simulink model "motor_rotation"  (R2022a)
settings: Solver=VariableStepAuto  StartTime=0.0  StopTime=10.0  RelTol=1e-3  AbsTol=1e-3
libraries: fl_lib x26, nesl_utility x11, ee_lib x4, slpidlib x2
settings Model: Creator=venka  LastModifiedBy=venka
settings SolverCC: AutoScaleAbsTol=off  AlgebraicLoopSolver=TrustRegion
settings DebuggingCC: UnconnectedInputMsg=warning  UnconnectedOutputMsg=warning  UnconnectedLineMsg=warning  SymbolicDimsDataTypeCodeGenerationDiagnostic=none  SFMachineParentedDataDiag=warning
settings SFSimCC: CustomCodeUndefinedFunction=UseInterfaceOnly
settings RTWCC: DLArmComputeVersion=19.05
settings SimscapeCC: SimscapeLogType=all  SimscapeLogSimulationStatistics=on  SimscapeLogDataHistory=10000

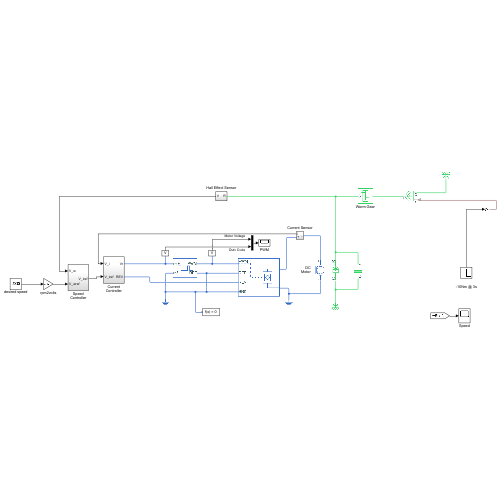
[thumbnail: Simulink's stored preview of the top-level diagram]
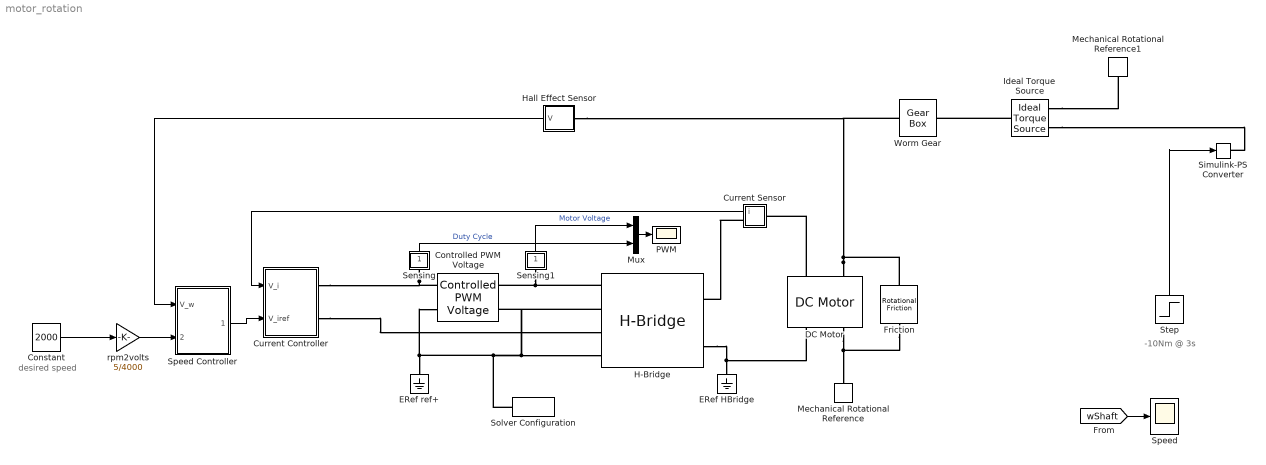
== system motor_rotation ==
  note: -10Nm @ 3s
  note: desired speed
  Constant : Constant  Value=2000
  Controlled PWM Voltage : ee_lib/Integrated Circuits/Controlled PWM Voltage  F=10000 Hz  TD=0 s  pulse_width_offset=0 s  pulse_min=0 s  pwm_or_av=2  event_type=1  sample_time=1e-6 s  Vmin=0 V  Vmax=5 V  Vm=5 V  u_min=0  u_max=1
  Current Controller : Subsystem
  Current Sensor : Subsystem
  DC Motor : ee_lib/Electromechanical/Brushed Motors/DC Motor  field_option=ee.enum.field_option.pm  Rf=100 Ohm  Lf=1 H  Laf=0.15 H  If0=0 A  parameterization=1  Ra=4.8 Ohm  La=1600e-6 H  emf_or_torque=2  Kv=0.0637 V/rpm  Ki=0.0637 N*m/A  T_stall=2.4e-4 N*m  w_max=1.91e+4 rpm  w_rated=1.5e+4 rpm  P_rated=0.08 W  V_rated=1.5 V  lam_param=1  i_noload=0 A  V_i_noload=1.5 V  J=2.5e-5 kg*m^2  lam=1e-08 N*m/(rad/s)  speed0=0 rpm  enable_fault_armature=simscape.enum.onoff.off  rev_faulted=1 / 3  G_faulted_armature=1e-5 S  fault_trigger_armature=ee.enum.faults.faultTrigger.temporal  t_fault_armature=1 s  max_permissible_current_armature=inf A  t_fail_on_current_armature=1 s  enable_fault_field=simscape.enum.onoff.off  G_faulted_field=1e-5 S  fault_trigger_field=ee.enum.faults.faultTrigger.temporal  t_fault_field=1 s  max_permissible_current_field=inf A  t_fail_on_current_field=1 s  fault_action=simscape.enum.assert.action.none  alpha=3.93e-3 1/K  Tmeas=25 degC  thermal_mass=100 J/K  initial_temperature=25 degC
  ERef HBridge : fl_lib/Electrical/Electrical Elements/Electrical Reference
      settings: SourceProductBaseCode=PW,SS,VE
  ERef ref+ : fl_lib/Electrical/Electrical Elements/Electrical Reference
      settings: SourceProductBaseCode=PW,SS,VE
  Friction : fl_lib/Mechanical/Rotational Elements/Rotational Friction  brkwy_trq=0.022 N*m  brkwy_vel=0.03347 rad/s  Col_trq=0.022 N*m  visc_coef=0 N*m/(rad/s)  w_specify=off  w_priority=High  w=0 rad/s  w_nominal_specify=off  w_nominal_unit=rad/s  w_nominal_value=1  t_specify=off  t_priority=High  t=0 N*m  t_nominal_specify=off  t_nominal_unit=N*m  t_nominal_value=1
      settings: SourceProductBaseCode=PW,SS,VE
  H-Bridge : ee_lib/Semiconductors & Converters/Converters/H-Bridge  supply_ports=ee.enum.supply_ports.hidesupply  pwm_or_av=ee.enum.pwm_or_av.averaged  regenerative_braking_mode=ee.enum.converters.regenerative_braking_mode.always_enabled  discontinuous=ee.enum.current_profile.continuous  freewheeling_mode=ee.enum.converters.freewheeling_mode.one_switch_one_diode  Rload=10 Ohm  Lload=1e-5 H  F=10 kHz  Venable=2.5 V  Vmax=5 V  Vreverse=2.5 V  Vbrake=2.5 V  Vm=24 V  Ron=0.1 Ohm  Don=0.1 Ohm  Goff=1e-6 S  Tmeas=298.15 K  Ron2=0.1 Ohm  Don2=0.05 Ohm  Tmeas2=398.15 K  thermal_mass=100 J/K  initial_temperature=298.15 K
  Hall Effect Sensor : Subsystem
  Ideal Torque Source : fl_lib/Mechanical/Mechanical Sources/Ideal Torque Source
      settings: SourceProductBaseCode=PW,SS,VE
  Mechanical Rotational Reference : fl_lib/Mechanical/Rotational Elements/Mechanical Rotational Reference
      settings: SourceProductBaseCode=PW,SS,VE
  Mechanical Rotational Reference1 : fl_lib/Mechanical/Rotational Elements/Mechanical Rotational Reference
      settings: SourceProductBaseCode=PW,SS,VE
  Mux : Mux  Inputs=2
  PWM : Scope
  Sensing : Subsystem
      mask Display: disp('V')
  Sensing1 : Subsystem
      mask Display: disp('V')
  Simulink-PS Converter : nesl_utility/Simulink-PS Converter  PhysicalDomain=network_engine_domain  SubClassName=ps_input  LeftPortType=input  RightPortType=output  PseudoPeriodic=off  Frequencies=[]  NoiseDistribution=none  NoiseParameters=[]  Unit=1  AffineConversion=off  FilteringAndDerivatives=provide  SimscapeFilterOrder=1  InputFilterTimeConstant=0.001  UdotUserProvided=0
      settings: SourceProductBaseCode=SS,PW,VE
  Solver Configuration : nesl_utility/Solver Configuration  PhysicalDomain=network_engine_domain  SubClassName=solver  LeftPortType=input  RightPortType=generic  Tones=[]  Harmonics=[]  SimulateNoise=off  Profile=off  UseLocalSampling=off  EnableSwitchedLinearOptims=on  FrequencyDomain=off  UseCCode=off  RelTol=0.001  AbsTol=1e-06  MinStep=1e-09  ToWorkspace=off  RevertToSquareIcSolve=off  NumHomotopyIterations=100  PhasorMode=off  PhasorModeNumHarmonics=1  IndexReductionMethod=DerivativeReplacement  DoDC=off  ResidualTolerance=1e-9  UseLocalSolver=off  LocalSolverChoice=NE_BACKWARD_EULER_ADVANCER  LocalSolverSampleTime=0.0001  DoFixedCost=off  MaxNonlinIter=3  MaxModeIter=2  ComputeImpulses=off  ImpulseIterations=2  LinearAlgebra=auto  LinearAlgebraNumThread=0  EquationFormulation=NE_TIME_EF  DelaysMemoryBudget=1024  AutomaticFiltering=on  FilteringTimeConstant=0.001  PartitionStorageMethod=AS_NEEDED  PartitionMemoryBudget=1024  PartitionMethod=FAST
      settings: SourceProductBaseCode=SS,PW,VE
  Speed : Scope
  Speed Controller : Subsystem
  Step : Step  Time=3  After=-10  SampleTime=0
  Worm Gear : fl_lib/Mechanical/Mechanisms/Gear Box  ratio=6.25  t_in_specify=off  t_in_priority=High  t_in=0 N*m  t_in_nominal_specify=off  t_in_nominal_unit=N*m  t_in_nominal_value=1  t_out_specify=off  t_out_priority=High  t_out=0 N*m  t_out_nominal_specify=off  t_out_nominal_unit=N*m  t_out_nominal_value=1
      settings: SourceProductBaseCode=PW,SS,VE
  rpm2volts : Gain  Gain=5/4000
  wires:
  Step/1 -> Simulink-PS Converter/1
  Mux/1 -> PWM/1
  Sensing/1(Out1) -> Mux/2  "Duty Cycle"
  Sensing1/1(Out1) -> Mux/1  "Motor Voltage"
  rpm2volts/1 -> Speed Controller/2(V_wref)
  Current Sensor/1(i) -> Current Controller/1(V_i)
  Constant/1 -> rpm2volts/1
  Hall Effect Sensor/1(V) -> Speed Controller/1(V_w)
  Speed Controller/1(V_iref) -> Current Controller/2(V_iref)
  [wShaft] -> Speed/1
  connections:
  Ideal Torque Source/RConn2 -- Mechanical Rotational Reference1/LConn1
  Ideal Torque Source/RConn1 -- Simulink-PS Converter/RConn1
  Solver Configuration/RConn1 -- ERef ref+/LConn1 -- Controlled PWM Voltage/LConn2 -- H-Bridge/LConn2 -- Controlled PWM Voltage/RConn2 -- H-Bridge/LConn4
  Sensing/LConn1 -- Controlled PWM Voltage/LConn1 -- Current Controller/RConn1
  ERef HBridge/LConn1 -- H-Bridge/RConn2 -- DC Motor/RConn1
  Friction/RConn1 -- Mechanical Rotational Reference/LConn1 -- DC Motor/RConn2
  Sensing1/LConn1 -- Controlled PWM Voltage/RConn1 -- H-Bridge/LConn1
  DC Motor/LConn2 -- Worm Gear/LConn1 -- Hall Effect Sensor/LConn1 -- Friction/LConn1
  Ideal Torque Source/LConn1 -- Worm Gear/RConn1
  Current Controller/RConn2 -- H-Bridge/LConn3
  DC Motor/LConn1 -- Current Sensor/LConn1
  Current Sensor/RConn1 -- H-Bridge/RConn1

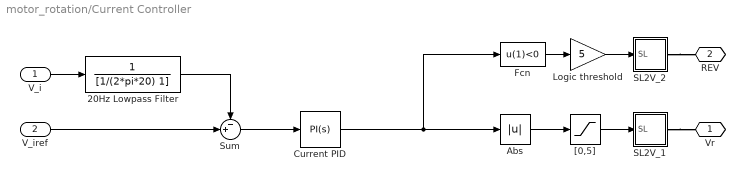
== system motor_rotation/Current Controller ==
  V_i : Inport
  V_iref : Inport  Port=2
  20Hz Lowpass Filter : TransferFcn  Denominator=[1/(2*pi*20) 1]
  Abs : Abs  SaturateOnIntegerOverflow=off
  Current PID : slpidlib/PID Controller  Controller=PI  Form=Parallel  TimeDomain=Continuous-time  UseExternalTs=off  SampleTime=-1  IntegratorMethod=Forward Euler  FilterMethod=Forward Euler  ControllerParametersSource=internal  P=1  I=50  UseKiTs=off  D=0  N=100  UseFilter=on  TunerSelectOption=Transfer Function Based (PID Tuner App)  InitialConditionSource=internal  InitialConditionForIntegrator=0  InitialConditionForFilter=0  DifferentiatorICPrevScaledInput=0  ExternalReset=none  TrackingMode=off  Kt=1  LimitOutput=off  SatLimitsSource=internal  UpperSaturationLimit=5  LowerSaturationLimit=-5  LinearizeAsGain=on  AntiWindupMode=back-calculation  Kb=1  POutMin=[]  POutMax=[]  IOutMin=[]  IOutMax=[]  DOutMin=[]  DOutMax=[]  NOutMin=[]  NOutMax=[]  SumOutMin=[]  SumOutMax=[]  SaturationOutMin=[]  SaturationOutMax=[]  PParamMin=[]  PParamMax=[]  IParamMin=[]  IParamMax=[]  DParamMin=[]  DParamMax=[]  NParamMin=[]  NParamMax=[]  KbParamMin=[]  KbParamMax=[]  KtParamMin=[]  KtParamMax=[]  KbOutMin=[]  KbOutMax=[]  KtOutMin=[]  KtOutMax=[]  IntegratorOutMin=[]  IntegratorOutMax=[]  FilterOutMin=[]  FilterOutMax=[]  SumI1OutMin=[]  SumI1OutMax=[]  SumI2OutMin=[]  SumI2OutMax=[]  SumI3OutMin=[]  SumI3OutMax=[]  SumI4OutMin=[]  SumI4OutMax=[]  SumDOutMin=[]  SumDOutMax=[]  DifferentiatorOutMin=[]  DifferentiatorOutMax=[]  FilterDiffOutCoefMin=[]  FilterDiffOutCoefMax=[]  ReciprocalOutMin=[]  ReciprocalOutMax=[]  SumDenOutMin=[]  SumDenOutMax=[]  SumNumOutMin=[]  SumNumOutMax=[]  DivideOutMin=[]  DivideOutMax=[]  UdiffTsProdOutMin=[]  UdiffTsProdOutMax=[]  NTsProdOutMin=[]  NTsProdOutMax=[]  UintegralTsProdOutMin=[]  UintegralTsProdOutMax=[]  UngainTsProdOutMin=[]  UngainTsProdOutMax=[]  IntegratorContinuousStateAttributes=''  IntegratorStateMustResolveToSignalObject=off  IntegratorRTWStateStorageClass=Auto  FilterContinuousStateAttributes=''  FilterStateMustResolveToSignalObject=off  FilterRTWStateStorageClass=Auto  ParallelPVariant=InternalParameters  IdealPVariant=Disabled  IVariant=InternalParameters  DVariant=Disabled  IntegratorVariant=Continuous  SatVariant=Disabled  AWVariant=Passthrough  PCopyVariant=Disabled  TRVariant=Disabled  FdbkBlocksVariant=Forward  IdealPFdbkVariant=Disabled  SatFdbkVariant=Disabled  DerivativeFilterVariant=Disabled  NVariant=Disabled  NCopyVariant=Disabled_SignalSpec  FilterICVariant=Disabled  IntegratorICVariant=InternalICs  ExternalResetVariant=Disabled  TRSumVariant=Passthrough  SumFdbkVariant=Disabled  SumVariant=Sum_PI  TsampFilterVariant=InternalTs  TsampNgainVariant=Passthrough  TsampIntegralVariant=Passthrough  ExternalSaturationOutDataTypeStr=Inherit: Same as second input  aMode=0
  Fcn : Fcn  Expr=u(1)<0
  Logic threshold : Gain  Gain=5
  SL2V_1 : Subsystem
  SL2V_2 : Subsystem
  Sum : Sum  Inputs=-+|
  "[0,5]" : Saturate  UpperLimit=5  LowerLimit=0
  Vr : PMIOPort  Side=Right
  REV : PMIOPort  Port=2  Side=Right
  wires:
  V_iref/1 -> Sum/2
  V_i/1 -> 20Hz Lowpass Filter/1
  20Hz Lowpass Filter/1 -> Sum/1
  Abs/1 -> "[0,5]"/1
  Fcn/1 -> Logic threshold/1
  Logic threshold/1 -> SL2V_2/1(SL)
  "[0,5]"/1 -> SL2V_1/1(SL)
  Current PID/1 -> Fcn/1, Abs/1
  Sum/1 -> Current PID/1
  connections:
  SL2V_1/RConn1 -- Vr/RConn1
  SL2V_2/RConn1 -- REV/RConn1

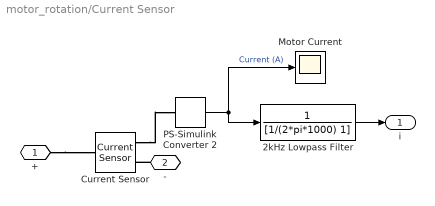
== system motor_rotation/Current Sensor ==
  2kHz Lowpass Filter : TransferFcn  Denominator=[1/(2*pi*1000) 1]
  Current Sensor : fl_lib/Electrical/Electrical Sensors/Current Sensor
      settings: SourceProductBaseCode=PW,SS,VE
  Motor Current : Scope
  PS-Simulink Converter 2 : nesl_utility/PS-Simulink Converter  PhysicalDomain=network_engine_domain  SubClassName=ps_output  LeftPortType=input  RightPortType=output  PseudoPeriodic=off  Frequencies=[]  VectorFormat=1-D array  Unit=A  AffineConversion=off
      settings: SourceProductBaseCode=SS,PW,VE
  + : PMIOPort  Side=Right
  - : PMIOPort  Port=2  Side=Left
  i : Outport  VectorParamsAs1DForOutWhenUnconnected=off
  wires:
  PS-Simulink Converter 2/1 -> 2kHz Lowpass Filter/1, Motor Current/1  "Current (A)"
  2kHz Lowpass Filter/1 -> i/1
  connections:
  +/RConn1 -- Current Sensor/LConn1
  -/RConn1 -- Current Sensor/RConn2
  Current Sensor/RConn1 -- PS-Simulink Converter 2/LConn1

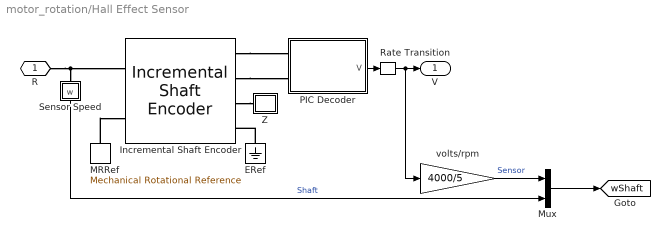
== system motor_rotation/Hall Effect Sensor ==
  ERef : fl_lib/Electrical/Electrical Elements/Electrical Reference
      settings: SourceProductBaseCode=PW,SS,VE
  Incremental Shaft Encoder : ee_lib/Sensors & Transducers/Incremental Shaft Encoder  NPulse=2  Vm=5 V  angle0=-1 deg
      settings: SourceProductBaseCode=PS  InternalSimscapePortConfiguration="{\"Bottom\":[],\"Left\":[{\"id\":\"R\",\"label\":\"R\",\"type\":\"foundation.mechanical.rotational.rotational\"},{\"id\":\"C\",\"label\":\"C\",\"type\":\"foundation.mechanical.rotational.rotational\"}],\"Right\":[{\"id\":\"A\",\"label\":\"A\",\"type\":\"foundation.electrical.electrical\"},{\"id\":\"B\",\"label\":\"B\",\"type\":\"foundation.electrical.electrical\"},{\"id\":\"Z\",\"label\":\"Z\",\"type\":\"foundation.electrical.electrical\"},{\"id\":\"GND\",\"label\":\"REF\",\"type\":\"foundation.electrical.electrical\"}],\"Top\":[]}"
  MRRef : fl_lib/Mechanical/Rotational Elements/Mechanical Rotational Reference
      settings: SourceProductBaseCode=PW,SS,VE
  Mux : Mux  Inputs=2
  PIC Decoder : Subsystem
  Rate Transition : RateTransition
  Sensor Speed : Subsystem
      mask Display: disp('w')
  Z : Subsystem
  volts/rpm : Gain  Gain=4000/5
  R : PMIOPort  Side=Left
  V : Outport  VectorParamsAs1DForOutWhenUnconnected=off
  tag scope: wShaft=global
  wires:
  PIC Decoder/1(V) -> Rate Transition/1
  Rate Transition/1 -> V/1, volts/rpm/1
  Mux/1 -> [wShaft]
  volts/rpm/1 -> Mux/1  "Sensor"
  Sensor Speed/1(w) -> Mux/2  "Shaft"
  connections:
  MRRef/LConn1 -- Incremental Shaft Encoder/LConn2
  R/RConn1 -- Incremental Shaft Encoder/LConn1 -- Sensor Speed/LConn1
  ERef/LConn1 -- Incremental Shaft Encoder/RConn4
  Incremental Shaft Encoder/RConn3 -- Z/LConn1
  Incremental Shaft Encoder/RConn1 -- PIC Decoder/LConn1
  Incremental Shaft Encoder/RConn2 -- PIC Decoder/LConn2

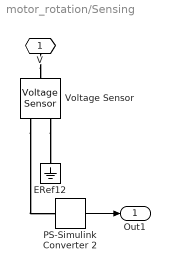
== system motor_rotation/Sensing ==
  ERef12 : fl_lib/Electrical/Electrical Elements/Electrical Reference
      settings: SourceProductBaseCode=PW,SS,VE
  PS-Simulink Converter 2 : nesl_utility/PS-Simulink Converter  PhysicalDomain=network_engine_domain  SubClassName=ps_output  LeftPortType=input  RightPortType=output  PseudoPeriodic=off  Frequencies=[]  VectorFormat=1-D array  Unit=V  AffineConversion=off
      settings: SourceProductBaseCode=SS,PW,VE
  Voltage Sensor : fl_lib/Electrical/Electrical Sensors/Voltage Sensor
      settings: SourceProductBaseCode=PW,SS,VE
  V : PMIOPort  Side=Left
  Out1 : Outport  VectorParamsAs1DForOutWhenUnconnected=off
  wires:
  PS-Simulink Converter 2/1 -> Out1/1
  connections:
  Voltage Sensor/RConn1 -- PS-Simulink Converter 2/LConn1
  Voltage Sensor/RConn2 -- ERef12/LConn1
  V/RConn1 -- Voltage Sensor/LConn1

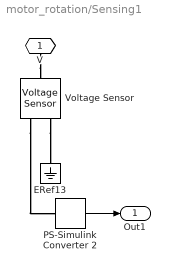
== system motor_rotation/Sensing1 ==
  ERef13 : fl_lib/Electrical/Electrical Elements/Electrical Reference
      settings: SourceProductBaseCode=PW,SS,VE
  PS-Simulink Converter 2 : nesl_utility/PS-Simulink Converter  PhysicalDomain=network_engine_domain  SubClassName=ps_output  LeftPortType=input  RightPortType=output  PseudoPeriodic=off  Frequencies=[]  VectorFormat=1-D array  Unit=V  AffineConversion=off
      settings: SourceProductBaseCode=SS,PW,VE
  Voltage Sensor : fl_lib/Electrical/Electrical Sensors/Voltage Sensor
      settings: SourceProductBaseCode=PW,SS,VE
  V : PMIOPort  Side=Left
  Out1 : Outport  VectorParamsAs1DForOutWhenUnconnected=off
  wires:
  PS-Simulink Converter 2/1 -> Out1/1
  connections:
  V/RConn1 -- Voltage Sensor/LConn1
  Voltage Sensor/RConn2 -- ERef13/LConn1
  Voltage Sensor/RConn1 -- PS-Simulink Converter 2/LConn1

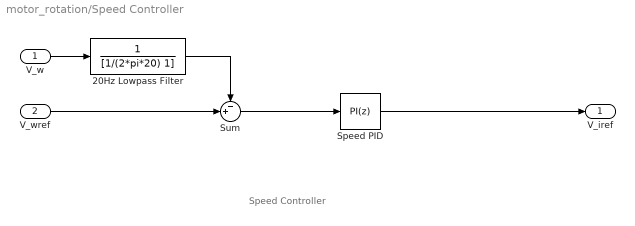
== system motor_rotation/Speed Controller ==
  note: Speed Controller
  V_w : Inport
  V_wref : Inport  Port=2
  20Hz Lowpass Filter : TransferFcn  Denominator=[1/(2*pi*20) 1]
  Speed PID : slpidlib/PID Controller  Controller=PI  Form=Parallel  TimeDomain=Discrete-time  UseExternalTs=off  SampleTime=0.01  IntegratorMethod=Forward Euler  FilterMethod=Forward Euler  ControllerParametersSource=internal  P=1  I=2  UseKiTs=off  D=0  N=100  UseFilter=on  TunerSelectOption=Transfer Function Based (PID Tuner App)  InitialConditionSource=internal  InitialConditionForIntegrator=0  InitialConditionForFilter=0  DifferentiatorICPrevScaledInput=0  ExternalReset=none  TrackingMode=off  Kt=1  LimitOutput=on  SatLimitsSource=internal  UpperSaturationLimit=5  LowerSaturationLimit=-5  LinearizeAsGain=on  AntiWindupMode=back-calculation  Kb=1  POutMin=[]  POutMax=[]  IOutMin=[]  IOutMax=[]  DOutMin=[]  DOutMax=[]  NOutMin=[]  NOutMax=[]  SumOutMin=[]  SumOutMax=[]  SaturationOutMin=[]  SaturationOutMax=[]  PParamMin=[]  PParamMax=[]  IParamMin=[]  IParamMax=[]  DParamMin=[]  DParamMax=[]  NParamMin=[]  NParamMax=[]  KbParamMin=[]  KbParamMax=[]  KtParamMin=[]  KtParamMax=[]  KbOutMin=[]  KbOutMax=[]  KtOutMin=[]  KtOutMax=[]  IntegratorOutMin=[]  IntegratorOutMax=[]  FilterOutMin=[]  FilterOutMax=[]  SumI1OutMin=[]  SumI1OutMax=[]  SumI2OutMin=[]  SumI2OutMax=[]  SumI3OutMin=[]  SumI3OutMax=[]  SumI4OutMin=[]  SumI4OutMax=[]  SumDOutMin=[]  SumDOutMax=[]  DifferentiatorOutMin=[]  DifferentiatorOutMax=[]  FilterDiffOutCoefMin=[]  FilterDiffOutCoefMax=[]  ReciprocalOutMin=[]  ReciprocalOutMax=[]  SumDenOutMin=[]  SumDenOutMax=[]  SumNumOutMin=[]  SumNumOutMax=[]  DivideOutMin=[]  DivideOutMax=[]  UdiffTsProdOutMin=[]  UdiffTsProdOutMax=[]  NTsProdOutMin=[]  NTsProdOutMax=[]  UintegralTsProdOutMin=[]  UintegralTsProdOutMax=[]  UngainTsProdOutMin=[]  UngainTsProdOutMax=[]  IntegratorContinuousStateAttributes=''  IntegratorStateMustResolveToSignalObject=off  IntegratorRTWStateStorageClass=Auto  FilterContinuousStateAttributes=''  FilterStateMustResolveToSignalObject=off  FilterRTWStateStorageClass=Auto  ParallelPVariant=InternalParameters  IdealPVariant=Disabled  IVariant=InternalParameters  DVariant=Disabled  IntegratorVariant=Discrete  SatVariant=Enabled  AWVariant=BackCalculation  PCopyVariant=Disabled  TRVariant=Disabled  FdbkBlocksVariant=Forward  IdealPFdbkVariant=Disabled  SatFdbkVariant=Disabled  DerivativeFilterVariant=Disabled  NVariant=Disabled  NCopyVariant=Disabled_SignalSpec  FilterICVariant=Disabled  IntegratorICVariant=InternalICs  ExternalResetVariant=Disabled  TRSumVariant=Passthrough  SumFdbkVariant=Disabled  SumVariant=Sum_PI  TsampFilterVariant=InternalTs  TsampNgainVariant=Passthrough  TsampIntegralVariant=Passthrough  ExternalSaturationOutDataTypeStr=Inherit: Same as second input  aMode=0
  Sum : Sum  Inputs=-+|
  V_iref : Outport  VectorParamsAs1DForOutWhenUnconnected=off
  wires:
  20Hz Lowpass Filter/1 -> Sum/1
  V_w/1 -> 20Hz Lowpass Filter/1
  V_wref/1 -> Sum/2
  Speed PID/1 -> V_iref/1
  Sum/1 -> Speed PID/1

== system motor_rotation/Current Controller/SL2V_1 ==
  SL : Inport
  Controlled Voltage Source : fl_lib/Electrical/Electrical Sources/Controlled Voltage Source
      settings: SourceProductBaseCode=PW,SS,VE
  Electrical Reference : fl_lib/Electrical/Electrical Elements/Electrical Reference
      settings: SourceProductBaseCode=PW,SS,VE
  Simulink-PS Converter : nesl_utility/Simulink-PS Converter  PhysicalDomain=network_engine_domain  SubClassName=ps_input  LeftPortType=input  RightPortType=output  PseudoPeriodic=off  Frequencies=[]  NoiseDistribution=none  NoiseParameters=[]  Unit=V  AffineConversion=off  FilteringAndDerivatives=zero  SimscapeFilterOrder=1  InputFilterTimeConstant=.001  UdotUserProvided=0
      settings: SourceProductBaseCode=SS,PW,VE
  V : PMIOPort  Side=Right
  wires:
  SL/1 -> Simulink-PS Converter/1
  connections:
  Electrical Reference/LConn1 -- Controlled Voltage Source/RConn2
  V/RConn1 -- Controlled Voltage Source/LConn1
  Simulink-PS Converter/RConn1 -- Controlled Voltage Source/RConn1

== system motor_rotation/Current Controller/SL2V_2 ==
  SL : Inport
  Controlled Voltage Source : fl_lib/Electrical/Electrical Sources/Controlled Voltage Source
      settings: SourceProductBaseCode=PW,SS,VE
  Electrical Reference : fl_lib/Electrical/Electrical Elements/Electrical Reference
      settings: SourceProductBaseCode=PW,SS,VE
  Simulink-PS Converter : nesl_utility/Simulink-PS Converter  PhysicalDomain=network_engine_domain  SubClassName=ps_input  LeftPortType=input  RightPortType=output  PseudoPeriodic=off  Frequencies=[]  NoiseDistribution=none  NoiseParameters=[]  Unit=V  AffineConversion=off  FilteringAndDerivatives=zero  SimscapeFilterOrder=1  InputFilterTimeConstant=.001  UdotUserProvided=0
      settings: SourceProductBaseCode=SS,PW,VE
  V : PMIOPort  Side=Right
  wires:
  SL/1 -> Simulink-PS Converter/1
  connections:
  Simulink-PS Converter/RConn1 -- Controlled Voltage Source/RConn1
  V/RConn1 -- Controlled Voltage Source/LConn1
  Electrical Reference/LConn1 -- Controlled Voltage Source/RConn2

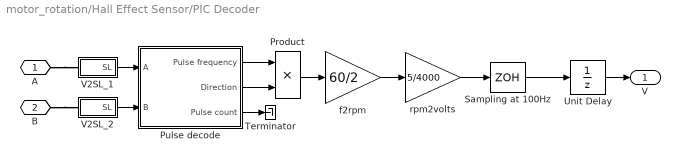
== system motor_rotation/Hall Effect Sensor/PIC Decoder ==
  Product : Product  RndMeth=Zero
  Pulse decode : Subsystem
  Sampling at 100Hz : ZeroOrderHold  SampleTime=0.01
  Terminator : Terminator
  Unit Delay : UnitDelay  SampleTime=0.01  HasFrameUpgradeWarning=on
  V2SL_1 : Subsystem
  V2SL_2 : Subsystem
  f2rpm : Gain  Gain=60/2
  rpm2volts : Gain  Gain=5/4000
  A : PMIOPort  Side=Left
  B : PMIOPort  Port=2  Side=Left
  V : Outport  VectorParamsAs1DForOutWhenUnconnected=off
  wires:
  Product/1 -> f2rpm/1
  Pulse decode/2(Direction) -> Product/2
  Pulse decode/1(Pulse frequency) -> Product/1
  Pulse decode/3(Pulse count) -> Terminator/1
  f2rpm/1 -> rpm2volts/1
  rpm2volts/1 -> Sampling at 100Hz/1
  V2SL_1/1(SL) -> Pulse decode/1(A)
  V2SL_2/1(SL) -> Pulse decode/2(B)
  Sampling at 100Hz/1 -> Unit Delay/1
  Unit Delay/1 -> V/1
  connections:
  A/RConn1 -- V2SL_1/LConn1
  B/RConn1 -- V2SL_2/LConn1

== system motor_rotation/Hall Effect Sensor/Sensor Speed ==
  MRRef5 : fl_lib/Mechanical/Rotational Elements/Mechanical Rotational Reference
      settings: SourceProductBaseCode=PW,SS,VE
  Motion Sensor : fl_lib/Mechanical/Mechanical Sensors/Ideal Rotational Motion Sensor  wrap_angle=simscape.enum.onoff.off  offset=0 rad
      settings: SourceProductBaseCode=PW,SS,VE
  PS-Simulink Converter 2 : nesl_utility/PS-Simulink Converter  PhysicalDomain=network_engine_domain  SubClassName=ps_output  LeftPortType=input  RightPortType=output  PseudoPeriodic=off  Frequencies=[]  VectorFormat=1-D array  Unit=rpm  AffineConversion=off
      settings: SourceProductBaseCode=SS,PW,VE
  R : PMIOPort  Side=Left
  w : Outport  VectorParamsAs1DForOutWhenUnconnected=off
  wires:
  PS-Simulink Converter 2/1 -> w/1
  connections:
  Motion Sensor/RConn2 -- PS-Simulink Converter 2/LConn1
  R/RConn1 -- Motion Sensor/LConn1
  MRRef5/LConn1 -- Motion Sensor/RConn1

== system motor_rotation/Hall Effect Sensor/Z ==
  ERef : fl_lib/Electrical/Electrical Elements/Electrical Reference
      settings: SourceProductBaseCode=PW,SS,VE
  PS-Simulink Converter 2 : nesl_utility/PS-Simulink Converter  PhysicalDomain=network_engine_domain  SubClassName=ps_output  LeftPortType=input  RightPortType=output  PseudoPeriodic=off  Frequencies=[]  VectorFormat=1-D array  Unit=V  AffineConversion=off
      settings: SourceProductBaseCode=SS,PW,VE
  Voltage Sensor : fl_lib/Electrical/Electrical Sensors/Voltage Sensor
      settings: SourceProductBaseCode=PW,SS,VE
  Vz : Scope
  u : PMIOPort  Side=Left
  wires:
  PS-Simulink Converter 2/1 -> Vz/1
  connections:
  Voltage Sensor/RConn2 -- ERef/LConn1
  Voltage Sensor/RConn1 -- PS-Simulink Converter 2/LConn1
  u/RConn1 -- Voltage Sensor/LConn1

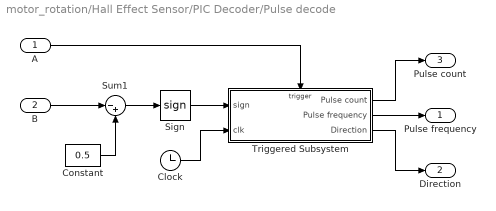
== system motor_rotation/Hall Effect Sensor/PIC Decoder/Pulse decode ==
  A : Inport
  B : Inport  Port=2
  Clock : Clock
  Constant : Constant  Value=0.5
  Sign : Signum
  Sum1 : Sum  Inputs=|-+
  Triggered Subsystem : Subsystem  TreatAsAtomicUnit=on
  Pulse frequency : Outport  VectorParamsAs1DForOutWhenUnconnected=off
  Direction : Outport  Port=2  VectorParamsAs1DForOutWhenUnconnected=off
  Pulse count : Outport  Port=3  VectorParamsAs1DForOutWhenUnconnected=off
  wires:
  Triggered Subsystem/3(Direction) -> Direction/1
  Triggered Subsystem/2(Pulse frequency) -> Pulse frequency/1
  Clock/1 -> Triggered Subsystem/2(clk)
  Triggered Subsystem/1(Pulse count) -> Pulse count/1
  A/1 -> Triggered Subsystem/Trigger
  Sign/1 -> Triggered Subsystem/1(sign)
  B/1 -> Sum1/1
  Sum1/1 -> Sign/1
  Constant/1 -> Sum1/2

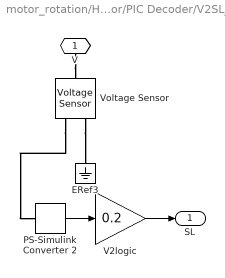
== system motor_rotation/Hall Effect Sensor/PIC Decoder/V2SL_1 ==
  ERef3 : fl_lib/Electrical/Electrical Elements/Electrical Reference
      settings: SourceProductBaseCode=PW,SS,VE
  PS-Simulink Converter 2 : nesl_utility/PS-Simulink Converter  PhysicalDomain=network_engine_domain  SubClassName=ps_output  LeftPortType=input  RightPortType=output  PseudoPeriodic=off  Frequencies=[]  VectorFormat=1-D array  Unit=V  AffineConversion=off
      settings: SourceProductBaseCode=SS,PW,VE
  V2logic : Gain  Gain=0.2
  Voltage Sensor : fl_lib/Electrical/Electrical Sensors/Voltage Sensor
      settings: SourceProductBaseCode=PW,SS,VE
  V : PMIOPort  Side=Left
  SL : Outport  VectorParamsAs1DForOutWhenUnconnected=off
  wires:
  PS-Simulink Converter 2/1 -> V2logic/1
  V2logic/1 -> SL/1
  connections:
  Voltage Sensor/RConn2 -- ERef3/LConn1
  V/RConn1 -- Voltage Sensor/LConn1
  Voltage Sensor/RConn1 -- PS-Simulink Converter 2/LConn1

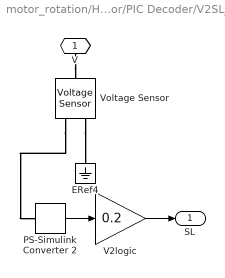
== system motor_rotation/Hall Effect Sensor/PIC Decoder/V2SL_2 ==
  ERef4 : fl_lib/Electrical/Electrical Elements/Electrical Reference
      settings: SourceProductBaseCode=PW,SS,VE
  PS-Simulink Converter 2 : nesl_utility/PS-Simulink Converter  PhysicalDomain=network_engine_domain  SubClassName=ps_output  LeftPortType=input  RightPortType=output  PseudoPeriodic=off  Frequencies=[]  VectorFormat=1-D array  Unit=V  AffineConversion=off
      settings: SourceProductBaseCode=SS,PW,VE
  V2logic : Gain  Gain=0.2
  Voltage Sensor : fl_lib/Electrical/Electrical Sensors/Voltage Sensor
      settings: SourceProductBaseCode=PW,SS,VE
  V : PMIOPort  Side=Left
  SL : Outport  VectorParamsAs1DForOutWhenUnconnected=off
  wires:
  V2logic/1 -> SL/1
  PS-Simulink Converter 2/1 -> V2logic/1
  connections:
  Voltage Sensor/RConn1 -- PS-Simulink Converter 2/LConn1
  V/RConn1 -- Voltage Sensor/LConn1
  Voltage Sensor/RConn2 -- ERef4/LConn1

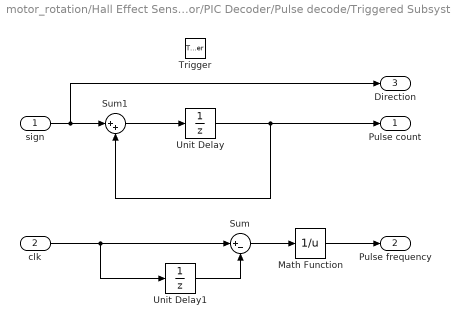
== system motor_rotation/Hall Effect Sensor/PIC Decoder/Pulse decode/Triggered Subsystem ==
  sign : Inport
  clk : Inport  Port=2
  Trigger : TriggerPort  VariantControl=Variant
  Math Function : Math  Operator=reciprocal  SignedPower=on
  Sum : Sum  Inputs=|+-
  Sum1 : Sum  Inputs=|++
  Unit Delay : UnitDelay  SampleTime=-1  HasFrameUpgradeWarning=on
  Unit Delay1 : UnitDelay  InitialCondition=-1e10  SampleTime=-1  HasFrameUpgradeWarning=on
  Pulse count : Outport  InitialOutput=0  VectorParamsAs1DForOutWhenUnconnected=off
  Pulse frequency : Outport  Port=2  VectorParamsAs1DForOutWhenUnconnected=off
  Direction : Outport  Port=3  InitialOutput=0  VectorParamsAs1DForOutWhenUnconnected=off
  wires:
  Math Function/1 -> Pulse frequency/1
  Sum/1 -> Math Function/1
  Unit Delay1/1 -> Sum/2
  clk/1 -> Sum/1, Unit Delay1/1
  Unit Delay/1 -> Sum1/2, Pulse count/1
  sign/1 -> Direction/1, Sum1/1
  Sum1/1 -> Unit Delay/1
